simulink model "sltestThrottlePositionActuatorMdlRef"  (R2023a)
settings: Solver=FixedStepDiscrete  StartTime=0.0  StopTime=10.0  FixedStep=0.005  RelTol=1e-3
PreLoadFcn:
  | HBridgeCmd_LkupTbl = Simulink.LookupTable;
  | HBridgeCmd_LkupTbl.Table.DataType = 'int16';
  | HBridgeCmd_LkupTbl.Table.FieldName = 'Table';
  | HBridgeCmd_LkupTbl.Table.Value = int16( ...
  |   [-2048 -1843 -1638 -1434 -1229 -1024 -819 -614 -410 -205 0 205 410 614 ...
  |    819 1024 1229 1434 1638 1843 2048]);
  | HBridgeCmd_LkupTbl.BreakpointsSpecification = 'Explicit values';
  | HBridgeCmd_LkupTbl.SupportTunableSize = false;
  | HBridgeCmd_LkupTbl.Breakpoints.DataType = 'single';
  | HBridgeCmd_LkupTbl.Breakpoints.FieldName = 'BP1';
  | HBridgeCmd_LkupTbl.Breakpoints.Value = ...
  |   [-100 -90 -80 -70 -60 -50 -40 -30 -20 -10 0 10 20 30 40 50 60 70 80 90 ...
  |    100];
  | HBridgeCmd_LkupTbl.Breakpoints.TunableSizeName = 'N1';
  | HBridgeCmd_LkupTbl.StructTypeInfo.Name = 'MyStruct_Actuator';
undefined symbols (not defined in the file): TPSPercentBkpt, TPSPercentTbl
settings Model: Creator=The MathWorks, Inc.  LastModifiedBy=The MathWorks, Inc.
settings SolverCC: AlgebraicLoopSolver=TrustRegion  MaxZcPerStep=1
settings DataIOCC: SaveFormat=StructureWithTime  ReturnWorkspaceOutputs=off
settings OptimizationCC: DefaultParameterBehavior=Inlined  PassReuseOutputArgsAs=Individual arguments  ZeroExternalMemoryAtStartup=off  ZeroInternalMemoryAtStartup=off  EfficientTunableParamExpr=on
settings DebuggingCC: ParameterTunabilityLossMsg=error  UnconnectedInputMsg=warning  UnconnectedOutputMsg=warning  UnconnectedLineMsg=warning  ArithmeticOperatorsInVariantConditions=warning
settings ModelReferenceCC: EnableRefExpFcnMdlSchedulingChecks=on
settings SFSimCC: SimUseLocalCustomCode=off  MATLABDynamicMemAlloc=off  CustomCodeUndefinedFunction=UseInterfaceOnly
settings RTWCC: Description=AUTOSAR  SystemTargetFile=autosar.tlc  GenCodeOnly=on  TemplateMakefile=ert_default_tmf  GenerateReport=on  RTWUseLocalCustomCode=off  IncludeHyperlinkInReport=on  LaunchReport=on  PortableWordSizes=on  GenerateTraceInfo=on  GenerateTraceReport=on  GenerateTraceReportSl=on  GenerateTraceReportSf=on  GenerateTraceReportEml=on  DLArmComputeVersion=19.05
settings CodeAppCC: ForceParamTrailComments=on  IgnoreCustomStorageClasses=off  OperatorAnnotations=on  SimulinkDataObjDesc=on  SFDataObjDesc=on  InsertBlockDesc=on
settings STFCustomTargetCC: MultiwordLength=256  ParMdlRefBuildCompliant=on  CompOptLevelCompliant=on  ConcurrentExecutionCompliant=off  IncludeMdlTerminateFcn=off  CombineOutputUpdateFcns=on  SuppressErrorStatus=on  ERTCustomFileBanners=on  SupportNonFinite=off  SupportComplex=off  SupportContinuousTime=off  SupportNonInlinedSFcns=off  RemoveResetFunc=on  MATLABClassNameForMDSCustomization=Simulink.SoftwareTarget.ERTCustomization  AutosarCompliant=on  GRTInterface=off  LookupTableObjectStructAxisOrder=2,1,3,4,...  LUTObjectStructOrderEvenSpacing=Size,Table,Breakpoints  SystemTargetFile=autosar.tlc
settings ERTTargetCC: TargetLangStandard=C99 (ISO)  ConcurrentExecutionCompliant=off  IncludeMdlTerminateFcn=off  SuppressErrorStatus=on  SupportNonFinite=off  SupportComplex=off  ModelStepFunctionPrototypeControlCompliant=off  CPPClassGenCompliant=off  AutosarCompliant=on  LookupTableObjectStructAxisOrder=2,1,3,4,...  LUTObjectStructOrderEvenSpacing=Size,Table,Breakpoints  InlinedParameterPlacement=NonHierarchical  ERTCustomFileTemplate=example_file_process.tlc

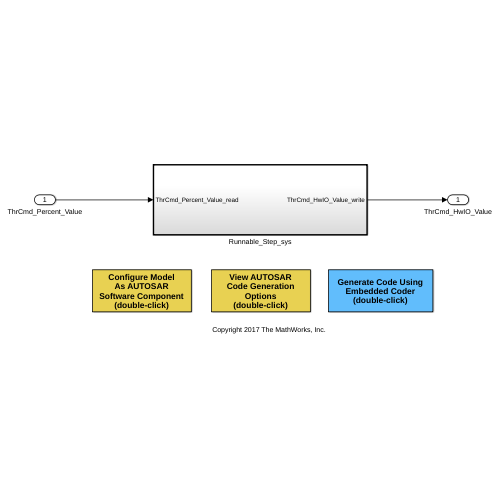
[thumbnail: Simulink's stored preview of the top-level diagram]
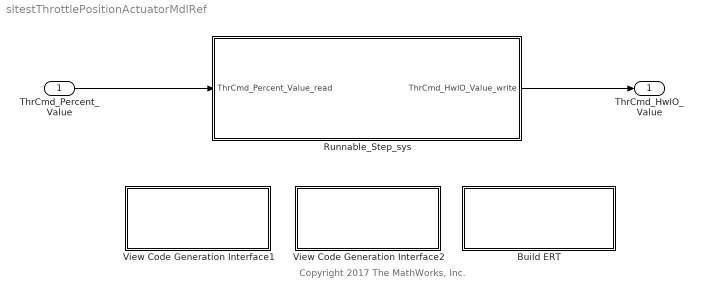
== system sltestThrottlePositionActuatorMdlRef ==
  note: Copyright 2017 The MathWorks, Inc.
  ThrCmd_Percent_Value : Inport  OutDataTypeStr=single  PortDimensions=1
  Build ERT : Subsystem  mask{attrib_overrides={'RTWCAPIParams','RTWCAPISignals','RTWCAPIStates'}}
      mask prompts: attrib_overrides "List of attributes to preserve (cell of strings):"
      mask help: Enter the attributes of the configuration set that you want preserved. Otherwise, the default configuration script will override your current settings.
      settings: OpenFcn=|
      | try
      |     if ~exist('rtwdemo_ert', 'dir')
      |         disp('Creating working directory rtwdemo_ert')
      |         mkdir('rtwdemo_ert')
      |     end
      |     cd('rtwdemo_ert');
      |     rtwbuilddemomodel(bdroot);
      |     cd('..');
      | catch myException
      |     rethrow(myException);
      | end
      mask Display:
      | disp(['Generate Code Using\n',...
      | 	 'Embedded Coder\n'...
      | 	  '(double-click)'])
  Runnable_Step_sys : Subsystem  TreatAsAtomicUnit=on  SystemSampleTime=0.005
  View Code Generation Interface1 : Subsystem
      settings: OpenFcn=autosar_ui_launch(bdroot)
      mask Display: disp('Configure Model\nAs AUTOSAR\nSoftware Component\n(double-click)')
  View Code Generation Interface2 : Subsystem
      settings: OpenFcn=|
      | dlg = slCfgPrmDlg(bdroot,'Open');
      | dlg = slCfgPrmDlg(bdroot,'TurnToPage',[message('RTW:configSet:configSetCodeGen').getString,'/',message('RTW:autosar:autosarCodeGenOptions').getString]);
      | clear dlg;
      mask Display: disp('View AUTOSAR\nCode Generation\nOptions\n(double-click)')
  ThrCmd_HwIO_Value : Outport  OutDataTypeStr=int16  PortDimensions=1  VectorParamsAs1DForOutWhenUnconnected=off
  wires:
  ThrCmd_Percent_Value/1 -> Runnable_Step_sys/1(ThrCmd_Percent_Value_read)
  Runnable_Step_sys/1(ThrCmd_HwIO_Value_write) -> ThrCmd_HwIO_Value/1

== system sltestThrottlePositionActuatorMdlRef/Build ERT ==

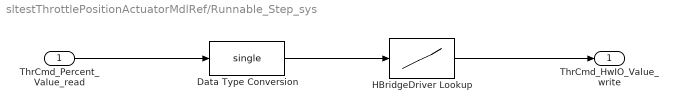
== system sltestThrottlePositionActuatorMdlRef/Runnable_Step_sys ==
  ThrCmd_Percent_Value_read : Inport
  Data Type Conversion : DataTypeConversion  OutDataTypeStr=single  SaturateOnIntegerOverflow=off  RndMeth=Floor
  HBridgeDriver Lookup : Lookup_n-D  NumberOfTableDimensions=1  DataSpecification=Lookup table object  LookupTableObject=HBridgeCmd_LkupTbl  BreakpointsForDimension1=TPSPercentBkpt  BreakpointsForDimension1DataTypeStr=single  IndexSearchMethod=Linear search  Table=TPSPercentTbl  TableDataTypeStr=single  InterpMethod=Nearest  InternalRulePriority=Speed  OutDataTypeStr=Inherit: Inherit from 'Table data'  RndMeth=Simplest
  ThrCmd_HwIO_Value_write : Outport  VectorParamsAs1DForOutWhenUnconnected=off
  wires:
  ThrCmd_Percent_Value_read/1 -> Data Type Conversion/1
  HBridgeDriver Lookup/1 -> ThrCmd_HwIO_Value_write/1
  Data Type Conversion/1 -> HBridgeDriver Lookup/1

== system sltestThrottlePositionActuatorMdlRef/View Code Generation Interface1 ==

== system sltestThrottlePositionActuatorMdlRef/View Code Generation Interface2 ==
